simulink model "Clark_Test"  (R2022a)
settings: Solver=VariableStepAuto  StartTime=0.0  StopTime=10.0  RelTol=1e-3
libraries: MyPMSMLibrary x1
settings Model: Creator=jff_1  LastModifiedBy=jff_1

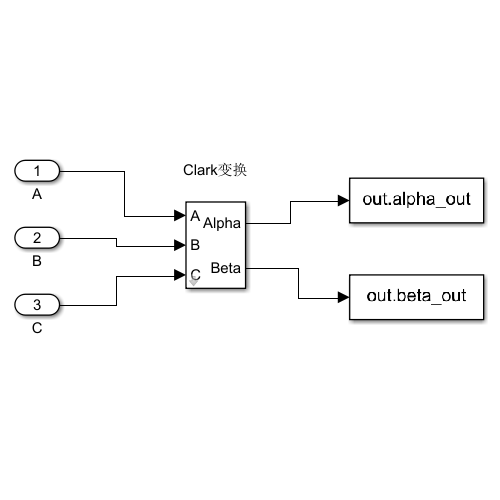
[thumbnail: Simulink's stored preview of the top-level diagram]
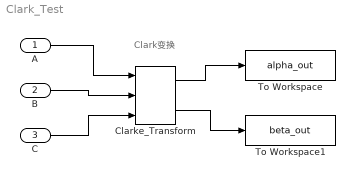
== system Clark_Test ==
  note: Clark变换
  A : Inport
  B : Inport  Port=2
  C : Inport  Port=3
  Clarke_Transform : MyPMSMLibrary/Transforms/Clarke_Transform
  To Workspace : ToWorkspace  VariableName=alpha_out  SampleTime=-1
  To Workspace1 : ToWorkspace  VariableName=beta_out  SampleTime=-1
  wires:
  Clarke_Transform/1 -> To Workspace/1
  Clarke_Transform/2 -> To Workspace1/1
  A/1 -> Clarke_Transform/1
  B/1 -> Clarke_Transform/2
  C/1 -> Clarke_Transform/3
